simulink subsystem "subsistema_mecanico"  (R2023b)
settings: Solver=VariableStepAuto  StartTime=0.0  StopTime=10.0  RelTol=1e-3
values from neighbouring files (symbols this model uses):
  b_eq = 2.1944e-5    (= 2.1944e-05)    [diagrama_polos_y_ceros_LTI.m]    (also in main.m = 2.19444444444e-05; parametros.m = 2.19444444444e-05)
  J_eq = 1.9785e-5    (= 1.9785e-05)    [diagrama_polos_y_ceros_LTI.m]    (also in main.m = 1.97847222222e-05; parametros.m = 1.97847222222e-05)
  k_l = 0.25    [main.m]    (also in parametros.m)
  r = 120.0    (= 120)    [diagrama_polos_y_ceros_LTI.m]    (also in main.m; parametros.m)
settings Model: Creator=nicol  LastModifiedBy=nicol

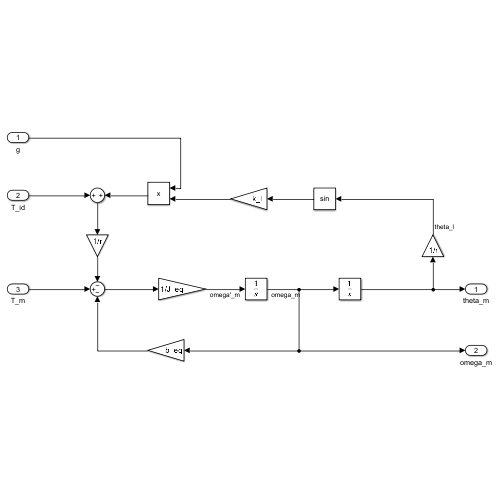
[thumbnail: Simulink's stored preview of the top-level diagram]
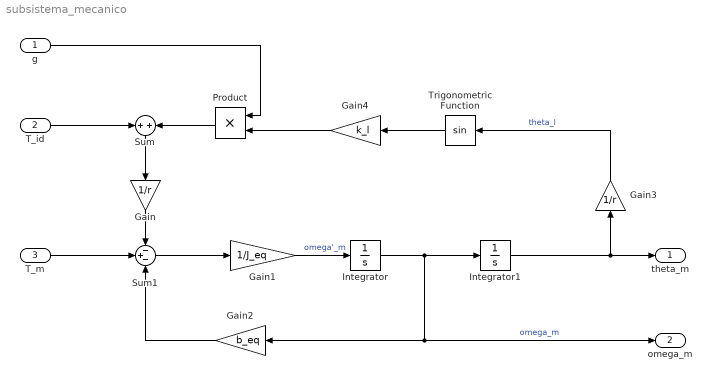
== system subsistema_mecanico ==
  g : Inport
  T_id : Inport  Port=2
  T_m : Inport  Port=3
  Gain : Gain  Gain=1/r
  Gain1 : Gain  Gain=1/J_eq
  Gain2 : Gain  Gain=b_eq
  Gain3 : Gain  Gain=1/r
  Gain4 : Gain  Gain=k_l
  Integrator : Integrator
  Integrator1 : Integrator
  Product : Product
  Sum : Sum
  Sum1 : Sum  Inputs=-+-
  Trigonometric Function : Trigonometry
  theta_m : Outport
  omega_m : Outport  Port=2
  wires:
  g/1 -> Product/1
  Product/1 -> Sum/2
  T_id/1 -> Sum/1
  Sum/1 -> Gain/1
  Gain/1 -> Sum1/1
  T_m/1 -> Sum1/2
  Sum1/1 -> Gain1/1
  Gain1/1 -> Integrator/1  "omega'_m"
  Integrator/1 -> Gain2/1, omega_m/1, Integrator1/1  "omega_m"
  Integrator1/1 -> Gain3/1, theta_m/1
  Gain2/1 -> Sum1/3
  Gain3/1 -> Trigonometric Function/1  "theta_l"
  Trigonometric Function/1 -> Gain4/1
  Gain4/1 -> Product/2
